simulink model "plant4_ester"  (R2025b)
settings: Solver=FixedStepAuto  StartTime=0.0  StopTime=10.0  RelTol=1e-3
values from neighbouring files (symbols this model uses):
  C12 = -(body.m*body.zb+2*mot.rot.m*mot.rot.zb)*wheel.r    [lab4_ester.m]
  den_LPF = [Tc, (Ts - Tc)]    [lab4_ester.m]
  dot_q0_sim = [0;0]    [lab4_ester.m]
  Fv1 = Fv + 2*gbox.N^2*mot.Kt*mot.Ke/mot.R *[1 -1; -1 1]    [lab4_ester.m]
  g2 = -(body.m*body.zb + 2*mot.rot.m*mot.rot.zb)*g    [lab4_ester.m]
  gam_ref = (positional_displacement/wheel.r)*rad2deg    [lab4_ester.m]
  K_lqr = K_e(2:5)    [lab4_ester.m]
  Ki = K_e(1)    [lab4_ester.m]
  M11 = 2*wheel.Iyy + 2*gbox.N^2*mot.rot.Iyy + (body.m + 2*wheel.m + 2*mot.rot.m)*wheel.r^2    [lab4_ester.m]
  M21_a = 2*gbox.N*(1-gbox.N)*mot.rot.Iyy    [lab4_ester.m]
  M21_b = (body.m*body.zb + 2*mot.rot.m*mot.rot.zb)*wheel.r    [lab4_ester.m]
  M22 = body.Iyy + 2*(1-gbox.N)^2*mot.rot.Iyy + body.m*body.zb^2 + 2*mot.rot.m*mot.rot.zb^2    [lab4_ester.m]
  Nu = N(5)    [lab4_ester.m]
  num_LPF = Ts    [lab4_ester.m]
  Nx = N(1:4)    [lab4_ester.m]
  q0_sim = [0; theta0_deg*deg2rad]    [lab4_ester.m]
  t_dist = 10    [lab4_ester.m]
  theta0_deg = 0    [lab4_ester.m]
  u_dist = 5/drv.duty2V    [lab4_ester.m]
  ua2tau1 = 2*gbox.N*mot.Kt/mot.R * [1; -1]    [lab4_ester.m]
undefined symbols (not defined in the file or in its folder): DiscIntNeverNeededParam, drv, g, gbox, ms22g, sens, Ts, wheel
settings Model: Creator=ester  LastModifiedBy=ester

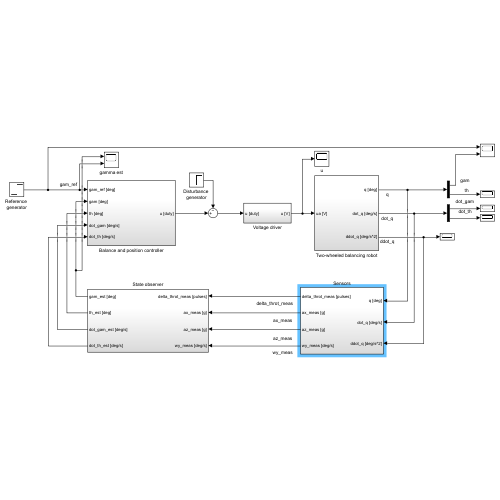
[thumbnail: Simulink's stored preview of the top-level diagram]
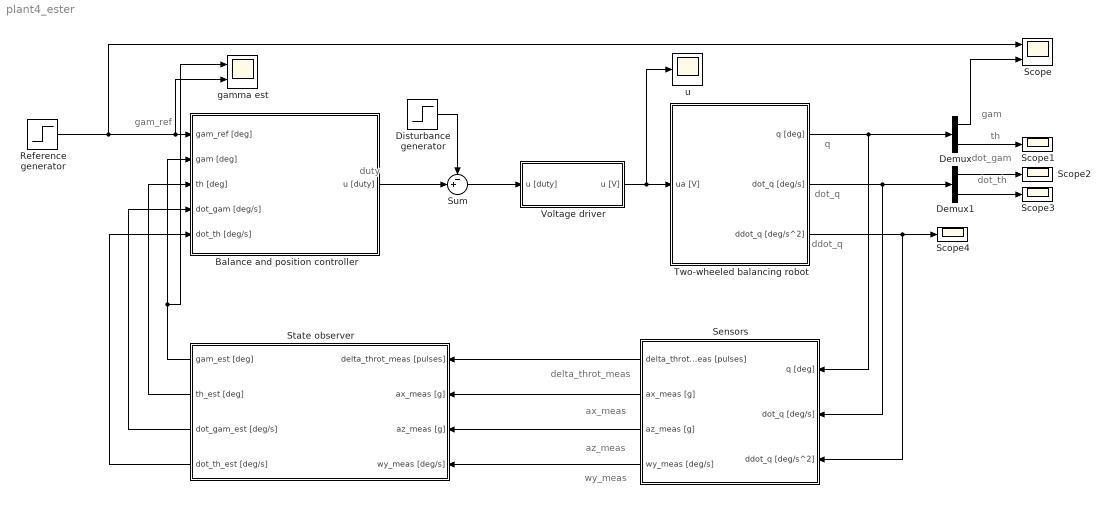
== system plant4_ester ==
  note: gam_ref
  note: ddot_q
  note: dot_q
  note: q
  note: dot_th
  note: dot_gam
  note: th
  note: gam
  note: duty
  note: ax_meas
  note: delta_throt_meas
  note: az_meas
  note: wy_meas
  Balance and position controller : Subsystem
  Demux : Demux  Outputs=2
  Demux1 : Demux  Outputs=2
  Disturbance generator : Step  Time=t_dist  After=u_dist  SampleTime=Ts
  Reference generator : Step  Time=0  After=gam_ref  SampleTime=Ts
  Scope : Scope  NumInputPorts=2
      settings: ActiveDisplayYMinimum=-418.6902528687242  ActiveDisplayYMaximum=65.245250159623708
  Scope{1..4} (4 alike) : Scope
      Scope1 settings: ActiveDisplayYMinimum=-1  ActiveDisplayYMaximum=1
      Scope2 settings: ActiveDisplayYMinimum=-1  ActiveDisplayYMaximum=1  DataLoggingVariableName=ScopeData2
      Scope3 settings: DataLoggingVariableName=ScopeData3
      Scope4 settings: ActiveDisplayYMinimum=-1  ActiveDisplayYMaximum=1  DataLoggingVariableName=ScopeData4
  Sensors : Subsystem
  State observer : Subsystem
  Sum : Sum  Inputs=-+|
  Two-wheeled balancing robot : Subsystem
  Voltage driver : Subsystem
  gamma est : Scope  NumInputPorts=2
      settings: ActiveDisplayYMinimum=-1  ActiveDisplayYMaximum=1  DataLoggingVariableName=ScopeData6
  u : Scope
      settings: DataLoggingVariableName=ScopeData5
  wires:
  Sum/1 -> Voltage driver/1(u [duty])
  Two-wheeled balancing robot/2(dot_q [deg/s]) -> Demux1/1, Sensors/2(dot_q [deg/s])
  Two-wheeled balancing robot/3(ddot_q [deg/s^2]) -> Scope4/1, Sensors/3(ddot_q [deg/s^2])
  Sensors/2(ax_meas [g]) -> State observer/2(ax_meas [g])
  Sensors/3(az_meas [g]) -> State observer/3(az_meas [g])
  Sensors/4(wy_meas [deg/s]) -> State observer/4(wy_meas [deg/s])
  Sensors/1(delta_throt_meas [pulses]) -> State observer/1(delta_throt_meas [pulses])
  Balance and position controller/1(u [duty]) -> Sum/2
  Two-wheeled balancing robot/1(q [deg]) -> Sensors/1(q [deg]), Demux/1
  Demux/1 -> Scope/2
  Demux/2 -> Scope1/1
  Demux1/2 -> Scope3/1
  Demux1/1 -> Scope2/1
  State observer/3(dot_gam_est [deg/s]) -> Balance and position controller/4(dot_gam [deg/s])
  State observer/4(dot_th_est [deg/s]) -> Balance and position controller/5(dot_th [deg/s])
  State observer/2(th_est [deg]) -> Balance and position controller/3(th [deg])
  State observer/1(gam_est [deg]) -> gamma est/1, Balance and position controller/2(gam [deg])
  Disturbance generator/1 -> Sum/1
  Reference generator/1 -> Scope/1, gamma est/2, Balance and position controller/1(gam_ref [deg])
  Voltage driver/1(u [V]) -> u/1, Two-wheeled balancing robot/1(ua [V])

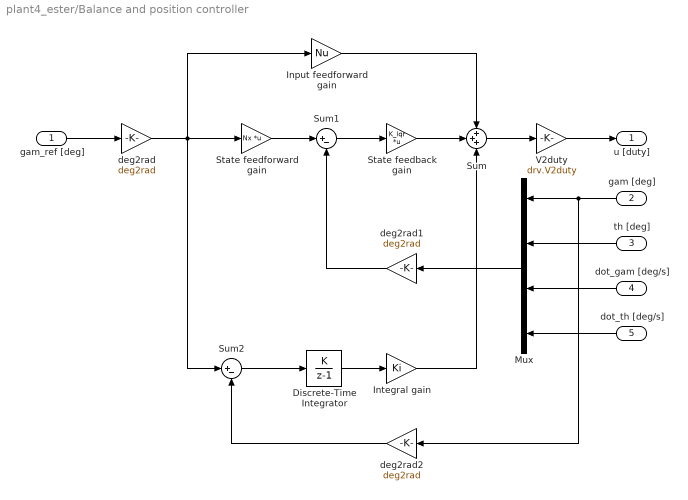
== system plant4_ester/Balance and position controller ==
  gam_ref [deg] : Inport
  gam [deg] : Inport  Port=2
  th [deg] : Inport  Port=3
  dot_gam [deg/s] : Inport  Port=4
  dot_th [deg/s] : Inport  Port=5
  Discrete-Time Integrator : DiscreteIntegrator  IntegratorMethod=Accumulation: Forward Euler  InitialCondition=theta0_deg*deg2rad  SampleTime=Ts  ICPrevOutput=DiscIntNeverNeededParam  ICPrevScaledInput=DiscIntNeverNeededParam
  Input feedforward gain : Gain  Gain=Nu
  Integral gain : Gain  Gain=Ki
  Mux : Mux
  State feedback gain : Gain  Gain=K_lqr  Multiplication=Matrix(K*u)
  State feedforward gain : Gain  Gain=Nx  Multiplication=Matrix(K*u)
  Sum : Sum  Inputs=+++
  Sum1 : Sum  Inputs=|+-
  Sum2 : Sum  Inputs=|+-
  V2duty : Gain  Gain=drv.V2duty
  deg2rad : Gain  Gain=deg2rad
  deg2rad1 : Gain  Gain=deg2rad
  deg2rad2 : Gain  Gain=deg2rad
  u [duty] : Outport
  wires:
  gam_ref [deg]/1 -> deg2rad/1
  deg2rad/1 -> Sum2/1, Input feedforward gain/1, State feedforward gain/1
  State feedback gain/1 -> Sum/2
  State feedforward gain/1 -> Sum1/1
  Sum1/1 -> State feedback gain/1
  Input feedforward gain/1 -> Sum/1
  Sum/1 -> V2duty/1
  V2duty/1 -> u [duty]/1
  gam [deg]/1 -> deg2rad2/1, Mux/1
  th [deg]/1 -> Mux/2
  dot_th [deg/s]/1 -> Mux/4
  dot_gam [deg/s]/1 -> Mux/3
  Mux/1 -> deg2rad1/1
  deg2rad1/1 -> Sum1/2
  Integral gain/1 -> Sum/3
  Sum2/1 -> Discrete-Time Integrator/1
  Discrete-Time Integrator/1 -> Integral gain/1
  deg2rad2/1 -> Sum2/2

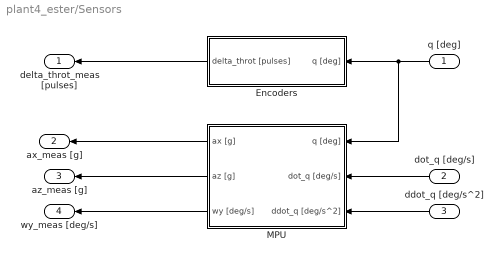
== system plant4_ester/Sensors ==
  q [deg] : Inport
  dot_q [deg/s] : Inport  Port=2
  ddot_q [deg/s^2] : Inport  Port=3
  Encoders : Subsystem
  MPU : Subsystem
  delta_throt_meas [pulses] : Outport
  ax_meas [g] : Outport  Port=2
  az_meas [g] : Outport  Port=3
  wy_meas [deg/s] : Outport  Port=4
  wires:
  q [deg]/1 -> Encoders/1(q [deg]), MPU/1(q [deg])
  Encoders/1(delta_throt [pulses]) -> delta_throt_meas [pulses]/1
  MPU/1(ax [g]) -> ax_meas [g]/1
  ddot_q [deg/s^2]/1 -> MPU/3(ddot_q [deg/s^2])
  dot_q [deg/s]/1 -> MPU/2(dot_q [deg/s])
  MPU/2(az [g]) -> az_meas [g]/1
  MPU/3(wy [deg/s]) -> wy_meas [deg/s]/1

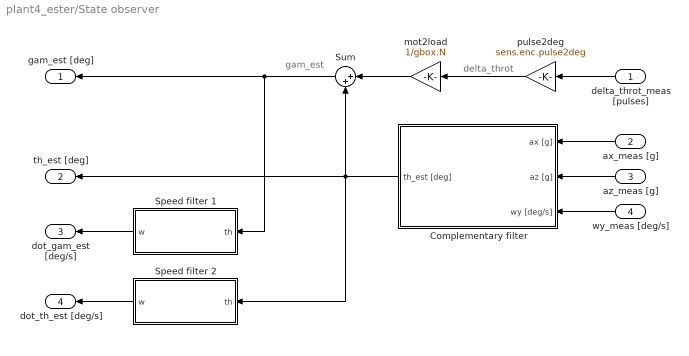
== system plant4_ester/State observer ==
  note: delta_throt
  note: gam_est
  delta_throt_meas [pulses] : Inport
  ax_meas [g] : Inport  Port=2
  az_meas [g] : Inport  Port=3
  wy_meas [deg/s] : Inport  Port=4
  Complementary filter : Subsystem
  Speed filter 1 : Subsystem
  Speed filter 2 : Subsystem
  Sum : Sum  Inputs=|++
  mot2load : Gain  Gain=1/gbox.N
  pulse2deg : Gain  Gain=sens.enc.pulse2deg
  gam_est [deg] : Outport
  th_est [deg] : Outport  Port=2
  dot_gam_est [deg/s] : Outport  Port=3
  dot_th_est [deg/s] : Outport  Port=4
  wires:
  pulse2deg/1 -> mot2load/1
  Speed filter 2/1(w) -> dot_th_est [deg/s]/1
  delta_throt_meas [pulses]/1 -> pulse2deg/1
  mot2load/1 -> Sum/1
  ax_meas [g]/1 -> Complementary filter/1(ax [g])
  Complementary filter/1(th_est [deg]) -> Speed filter 2/1(th), th_est [deg]/1, Sum/2
  Sum/1 -> gam_est [deg]/1, Speed filter 1/1(th)
  Speed filter 1/1(w) -> dot_gam_est [deg/s]/1
  az_meas [g]/1 -> Complementary filter/2(az [g])
  wy_meas [deg/s]/1 -> Complementary filter/3(wy [deg/s])

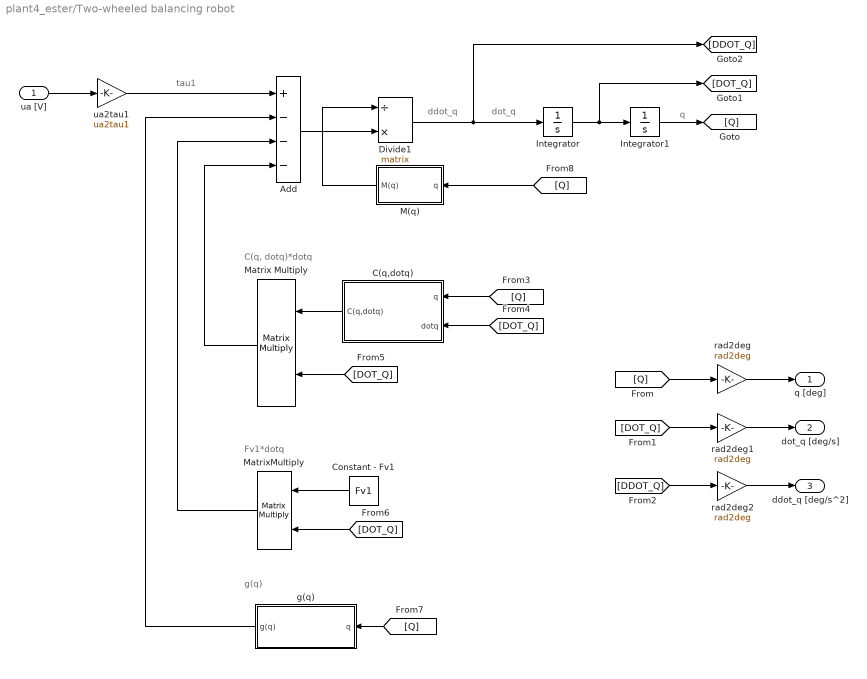
== system plant4_ester/Two-wheeled balancing robot ==
  note: q
  note: dot_q
  note: ddot_q
  note: tau1
  note: g(q)
  note: Fv1*dotq
  note: C(q, dotq)*dotq
  ua [V] : Inport
  "Add " : Sum  Inputs=+---
  C(q,dotq) : Subsystem
      mask Display: color('red');
  Constant - Fv1 : Constant  Value=Fv1
  Divide1 : Product  Inputs=/*  Multiplication=Matrix(*)
  "Integrator " : Integrator  InitialCondition=dot_q0_sim
  "Integrator1 " : Integrator  InitialCondition=q0_sim
  M(q) : Subsystem
  Matrix Multiply : Product  Multiplication=Matrix(*)
  MatrixMultiply : Product  Multiplication=Matrix(*)
  g(q) : Subsystem
  rad2deg : Gain  Gain=rad2deg
  rad2deg1 : Gain  Gain=rad2deg
  rad2deg2 : Gain  Gain=rad2deg
  ua2tau1 : Gain  Gain=ua2tau1
  q [deg] : Outport
  dot_q [deg/s] : Outport  Port=2
  ddot_q [deg/s^2] : Outport  Port=3
  wires:
  [DOT_Q] -> MatrixMultiply/2
  MatrixMultiply/1 -> "Add "/3
  [DOT_Q] -> C(q,dotq)/2(dotq)
  [Q] -> M(q)/1(q)
  [DOT_Q] -> Matrix Multiply/2
  [DDOT_Q] -> rad2deg2/1
  rad2deg2/1 -> ddot_q [deg/s^2]/1
  "Integrator1 "/1 -> [Q]
  [DOT_Q] -> rad2deg1/1
  [Q] -> g(q)/1(q)
  rad2deg/1 -> q [deg]/1
  [Q] -> rad2deg/1
  Constant - Fv1/1 -> MatrixMultiply/1
  Divide1/1 -> "Integrator "/1, [DDOT_Q]
  g(q)/1(g(q)) -> "Add "/2
  "Add "/1 -> Divide1/2
  ua [V]/1 -> ua2tau1/1
  C(q,dotq)/1(C(q,dotq)) -> Matrix Multiply/1
  ua2tau1/1 -> "Add "/1
  Matrix Multiply/1 -> "Add "/4
  [Q] -> C(q,dotq)/1(q)
  rad2deg1/1 -> dot_q [deg/s]/1
  "Integrator "/1 -> "Integrator1 "/1, [DOT_Q]
  M(q)/1(M(q)) -> Divide1/1

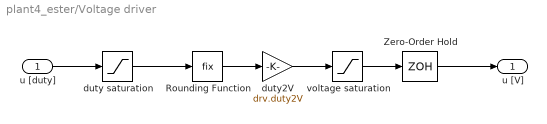
== system plant4_ester/Voltage driver ==
  u [duty] : Inport
  Rounding Function : Rounding  Operator=fix
  "Zero-Order Hold " : ZeroOrderHold  SampleTime=Ts
  duty saturation : Saturate  UpperLimit=drv.dutymax  LowerLimit=-drv.dutymax
  duty2V : Gain  Gain=drv.duty2V
  voltage saturation : Saturate  UpperLimit=drv.Vbus  LowerLimit=-drv.Vbus
  u [V] : Outport
  wires:
  u [duty]/1 -> duty saturation/1
  "Zero-Order Hold "/1 -> u [V]/1
  voltage saturation/1 -> "Zero-Order Hold "/1
  duty2V/1 -> voltage saturation/1
  Rounding Function/1 -> duty2V/1
  duty saturation/1 -> Rounding Function/1

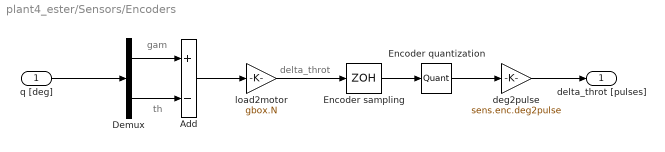
== system plant4_ester/Sensors/Encoders ==
  note: delta_throt
  note: th
  note: gam
  q [deg] : Inport
  Add : Sum  Inputs=+-
  Demux : Demux  Outputs=2
  Encoder quantization : Quantizer  QuantizationInterval=sens.enc.pulse2deg
  Encoder sampling : ZeroOrderHold  SampleTime=Ts
  deg2pulse : Gain  Gain=sens.enc.deg2pulse
  load2motor : Gain  Gain=gbox.N
  delta_throt [pulses] : Outport
  wires:
  q [deg]/1 -> Demux/1
  Demux/1 -> Add/1
  Demux/2 -> Add/2
  Add/1 -> load2motor/1
  load2motor/1 -> Encoder sampling/1
  Encoder sampling/1 -> Encoder quantization/1
  Encoder quantization/1 -> deg2pulse/1
  deg2pulse/1 -> delta_throt [pulses]/1

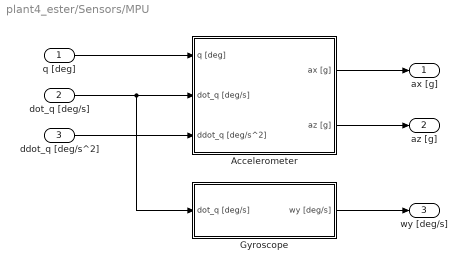
== system plant4_ester/Sensors/MPU ==
  q [deg] : Inport
  dot_q [deg/s] : Inport  Port=2
  ddot_q [deg/s^2] : Inport  Port=3
  Accelerometer : Subsystem
  Gyroscope : Subsystem
  ax [g] : Outport
  az [g] : Outport  Port=2
  wy [deg/s] : Outport  Port=3
  wires:
  q [deg]/1 -> Accelerometer/1(q [deg])
  dot_q [deg/s]/1 -> Gyroscope/1(dot_q [deg/s]), Accelerometer/2(dot_q [deg/s])
  ddot_q [deg/s^2]/1 -> Accelerometer/3(ddot_q [deg/s^2])
  Accelerometer/1(ax [g]) -> ax [g]/1
  Accelerometer/2(az [g]) -> az [g]/1
  Gyroscope/1(wy [deg/s]) -> wy [deg/s]/1

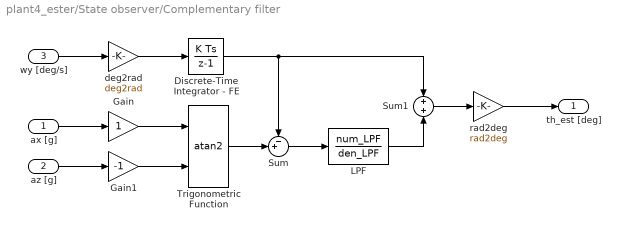
== system plant4_ester/State observer/Complementary filter ==
  ax [g] : Inport
  az [g] : Inport  Port=2
  wy [deg/s] : Inport  Port=3
  Discrete-Time Integrator - FE : DiscreteIntegrator  InitialCondition=theta0_deg*deg2rad  SampleTime=Ts  ICPrevOutput=DiscIntNeverNeededParam  ICPrevScaledInput=DiscIntNeverNeededParam
  Gain : Gain
  Gain1 : Gain  Gain=-1
  LPF : TransferFcn  Numerator=num_LPF  Denominator=den_LPF
  Sum : Sum  Inputs=-+|
  Sum1 : Sum
  "Trigonometric Function " : Trigonometry  Operator=atan2
  deg2rad : Gain  Gain=deg2rad
  rad2deg : Gain  Gain=rad2deg
  th_est [deg] : Outport
  wires:
  Sum/1 -> LPF/1
  Gain1/1 -> "Trigonometric Function "/2
  deg2rad/1 -> Discrete-Time Integrator - FE/1
  LPF/1 -> Sum1/2
  "Trigonometric Function "/1 -> Sum/2
  Discrete-Time Integrator - FE/1 -> Sum1/1, Sum/1
  Sum1/1 -> rad2deg/1
  Gain/1 -> "Trigonometric Function "/1
  rad2deg/1 -> th_est [deg]/1
  az [g]/1 -> Gain1/1
  wy [deg/s]/1 -> deg2rad/1
  ax [g]/1 -> Gain/1

== system plant4_ester/State observer/Speed filter 1 ==
  th : Inport
  Discrete Transfer Fcn : DiscreteTransferFcn  Numerator=[1 0 0 -1]  Denominator=[3*Ts 0 0 0]
  w : Outport
  wires:
  th/1 -> Discrete Transfer Fcn/1
  Discrete Transfer Fcn/1 -> w/1

== system plant4_ester/State observer/Speed filter 2 ==
  th : Inport
  Discrete Transfer Fcn : DiscreteTransferFcn  Numerator=[1 0 0 -1]  Denominator=[3*Ts 0 0 0]
  w : Outport
  wires:
  th/1 -> Discrete Transfer Fcn/1
  Discrete Transfer Fcn/1 -> w/1

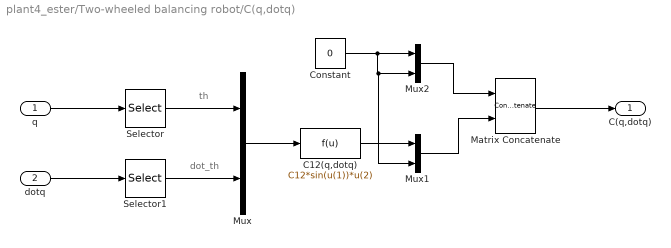
== system plant4_ester/Two-wheeled balancing robot/C(q,dotq) ==
  note: th
  note: dot_th
  q : Inport
  dotq : Inport  Port=2
  C12(q,dotq) : Fcn  Expr=C12*sin(u(1))*u(2)
  Constant : Constant  Value=0
  Matrix Concatenate : Concatenate  Mode=Multidimensional array  ConcatenateDimension=2
  Mux : Mux  Inputs=2
  Mux1 : Mux  Inputs=2
  Mux2 : Mux  Inputs=2
  Selector : Selector  InputPortWidth=2  IndexOptions=Index vector (dialog)  Indices=2  OutputSizes=1
  Selector1 : Selector  InputPortWidth=2  IndexOptions=Index vector (dialog)  Indices=2  OutputSizes=1
  C(q,dotq) : Outport
  wires:
  q/1 -> Selector/1
  Selector/1 -> Mux/1
  dotq/1 -> Selector1/1
  Selector1/1 -> Mux/2
  Mux/1 -> C12(q,dotq)/1
  C12(q,dotq)/1 -> Mux1/1
  Constant/1 -> Mux1/2, Mux2/2, Mux2/1
  Mux2/1 -> Matrix Concatenate/1
  Mux1/1 -> Matrix Concatenate/2
  Matrix Concatenate/1 -> C(q,dotq)/1

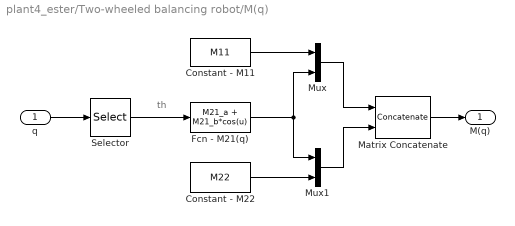
== system plant4_ester/Two-wheeled balancing robot/M(q) ==
  note: th
  q : Inport
  Constant - M11 : Constant  Value=M11
  Constant - M22 : Constant  Value=M22
  Fcn - M21(q) : Fcn  Expr=M21_a + M21_b*cos(u)
  Matrix Concatenate : Concatenate  Mode=Multidimensional array  ConcatenateDimension=2
  Mux : Mux  Inputs=2
  Mux1 : Mux  Inputs=2
  Selector : Selector  InputPortWidth=2  IndexOptions=Index vector (dialog)  Indices=2  OutputSizes=1
  M(q) : Outport
  wires:
  q/1 -> Selector/1
  Selector/1 -> Fcn - M21(q)/1
  Fcn - M21(q)/1 -> Mux1/1, Mux/2
  Constant - M11/1 -> Mux/1
  Mux/1 -> Matrix Concatenate/1
  Mux1/1 -> Matrix Concatenate/2
  Matrix Concatenate/1 -> M(q)/1
  Constant - M22/1 -> Mux1/2

== system plant4_ester/Two-wheeled balancing robot/g(q) ==
  note: th
  q : Inport
  Constant - g1 : Constant  Value=0
  Fcn - g2(q) : Fcn  Expr=g2*sin(u)
  Mux : Mux  Inputs=2
  Selector : Selector  InputPortWidth=2  IndexOptions=Index vector (dialog)  Indices=2  OutputSizes=1
  g(q) : Outport
  wires:
  q/1 -> Selector/1
  Selector/1 -> Fcn - g2(q)/1
  Fcn - g2(q)/1 -> Mux/2
  Mux/1 -> g(q)/1
  Constant - g1/1 -> Mux/1

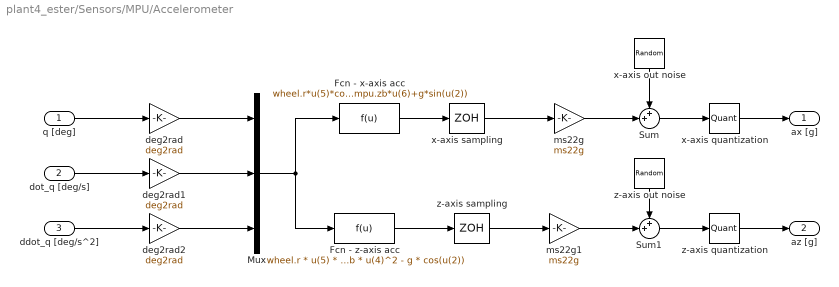
== system plant4_ester/Sensors/MPU/Accelerometer ==
  q [deg] : Inport
  dot_q [deg/s] : Inport  Port=2
  ddot_q [deg/s^2] : Inport  Port=3
  Fcn - x-axis acc : Fcn  Expr=wheel.r*u(5)*cos(u(2))+sens.mpu.zb*u(6)+g*sin(u(2))
  Fcn - z-axis acc : Fcn  Expr=wheel.r * u(5) * sin(u(2)) - sens.mpu.zb * u(4)^2 - g * cos(u(2))
  Mux : Mux  Inputs=3
  Sum : Sum  Inputs=++|
  Sum1 : Sum  Inputs=++|
  deg2rad : Gain  Gain=deg2rad
  deg2rad1 : Gain  Gain=deg2rad
  deg2rad2 : Gain  Gain=deg2rad
  ms22g : Gain  Gain=ms22g
  ms22g1 : Gain  Gain=ms22g
  x-axis out noise : RandomNumber  Variance=sens.mpu.acc.noisevar  SampleTime=Ts
  x-axis quantization : Quantizer  QuantizationInterval=sens.mpu.acc.LSB2g
  x-axis sampling : ZeroOrderHold  SampleTime=Ts
  z-axis out noise : RandomNumber  Variance=sens.mpu.acc.noisevar  SampleTime=Ts
  z-axis quantization : Quantizer  QuantizationInterval=sens.mpu.acc.LSB2g
  z-axis sampling : ZeroOrderHold  SampleTime=Ts
  ax [g] : Outport
  az [g] : Outport  Port=2
  wires:
  dot_q [deg/s]/1 -> deg2rad1/1
  q [deg]/1 -> deg2rad/1
  ddot_q [deg/s^2]/1 -> deg2rad2/1
  deg2rad1/1 -> Mux/2
  deg2rad/1 -> Mux/1
  deg2rad2/1 -> Mux/3
  Mux/1 -> Fcn - z-axis acc/1, Fcn - x-axis acc/1
  Fcn - x-axis acc/1 -> x-axis sampling/1
  Fcn - z-axis acc/1 -> z-axis sampling/1
  x-axis sampling/1 -> ms22g/1
  z-axis sampling/1 -> ms22g1/1
  ms22g/1 -> Sum/2
  x-axis out noise/1 -> Sum/1
  z-axis out noise/1 -> Sum1/1
  ms22g1/1 -> Sum1/2
  Sum1/1 -> z-axis quantization/1
  z-axis quantization/1 -> az [g]/1
  Sum/1 -> x-axis quantization/1
  x-axis quantization/1 -> ax [g]/1

== system plant4_ester/Sensors/MPU/Gyroscope ==
  dot_q [deg/s] : Inport
  "Random Number " : RandomNumber  Variance=sens.mpu.gyro.noisevar  SampleTime=Ts
  "Selector " : Selector  InputPortWidth=2  IndexOptions=Index vector (dialog)  Indices=2  OutputSizes=1
  Sum : Sum  Inputs=++|
  y-axis ampling : ZeroOrderHold  SampleTime=Ts
  y-axis quantizer : Quantizer  QuantizationInterval=sens.mpu.gyro.LSB2degs
  wy [deg/s] : Outport
  wires:
  dot_q [deg/s]/1 -> "Selector "/1
  "Selector "/1 -> y-axis ampling/1
  y-axis ampling/1 -> Sum/2
  "Random Number "/1 -> Sum/1
  Sum/1 -> y-axis quantizer/1
  y-axis quantizer/1 -> wy [deg/s]/1
